simulink model "half_subtractor"  (R2021a)
settings: Solver=VariableStepAuto  StartTime=0.0  StopTime=10.0  RelTol=1e-3
settings Model: Creator=kbhar  LastModifiedBy=kbhar

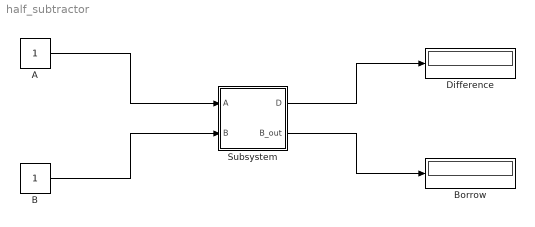
== system half_subtractor ==
  A : Constant
  B : Constant
  Borrow : Display
  Difference : Display
  Subsystem : Subsystem
  wires:
  A/1 -> Subsystem/1(A)
  B/1 -> Subsystem/2(B)
  Subsystem/1(D) -> Difference/1
  Subsystem/2(B_out) -> Borrow/1

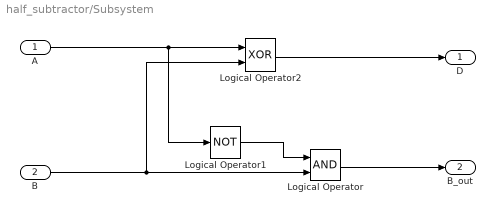
== system half_subtractor/Subsystem ==
  A : Inport
  B : Inport  Port=2
  Logical Operator : Logic  AllPortsSameDT=off  OutDataTypeStr=boolean
  Logical Operator1 : Logic  Operator=NOT  AllPortsSameDT=off  OutDataTypeStr=boolean
  Logical Operator2 : Logic  Operator=XOR  AllPortsSameDT=off  OutDataTypeStr=boolean
  D : Outport
  B_out : Outport  Port=2
  wires:
  B/1 -> Logical Operator/2, Logical Operator2/2
  A/1 -> Logical Operator2/1, Logical Operator1/1
  Logical Operator1/1 -> Logical Operator/1
  Logical Operator2/1 -> D/1
  Logical Operator/1 -> B_out/1
